simulink model "bh_6dof_NEWTON_explore_DRAG"  (R2017a)
settings: Solver=ode23t  StartTime=0.0  StopTime=200  FixedStep=0.001  RelTol=1e-5  EnableMultiTasking=on
undefined symbols (not defined in the file or in its folder): P_elec, P_mot, P_one_prop, P_rot, P_veh, sigbuilder_block
libraries: bh_6dof_LIBRARY x47, simulink x28, simulink_extras x25
(part 4 of 4)

== matlab function bh_6dof_NEWTON_explore_DRAG/CONT_SYS W_MOT_CMDS1/w2toFM ==
  data: L input; Thrust output; Thrust_const input; Twist_const input; w2_col input; TQ_roll_X output; TQ_pit_Y output; TQ_yaw_Z output
function [Thrust, TQ_roll_X, TQ_pit_Y, TQ_yaw_Z] = w2toFM(L, Thrust_const, Twist_const, w2_col)
%#codegen

    % simplify the variable names
    b = Thrust_const;
    k = Twist_const;

    % construct the co-efficient matrix:
    %  F_and_M = C * w^2
    
    C = [     b,    b,    b,    b;
              0,    b*L,  0,   -b*L;
             -b*L,  0,    b*L,  0;
             -k,    k,   -k,    k; ];

    % solve for the FM_col
    %   FM_col = [Thrust, TQ_roll_X, TQ_pit_Y, TQ_yaw_Z].' ;
    
    FM_col  =  C * w2_col;
    
    Thrust    =  FM_col(1);
    TQ_roll_X =  FM_col(2);
    TQ_pit_Y  =  FM_col(3);
    TQ_yaw_Z  =  FM_col(4);
    
end

== matlab function bh_6dof_NEWTON_explore_DRAG/Construct_DRAG_vec/aero_DRAG/UNIT_VEL_VEC ==
  data: v input; unit_v output
function unit_v = fcn(v)

% create unit velocity vector
the_MAG = norm(v);

unit_v = v;

% check for the [0,0,0] case
if(the_MAG > 0.001)
    unit_v = unit_v/the_MAG;
end

end
